simulink subsystem "encodersZ"  (R2023b)
settings: Solver=VariableStepAuto  StartTime=0.0  StopTime=10.0  RelTol=1e-3
libraries: arduinosensorlib x2, simulink x1
settings Model: Creator=Carlos  LastModifiedBy=Carlos

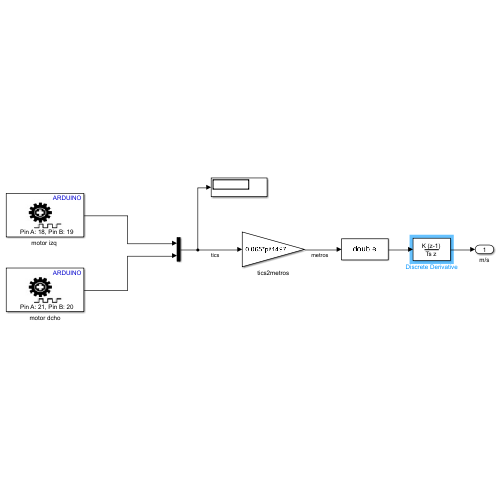
[thumbnail: Simulink's stored preview of the top-level diagram]
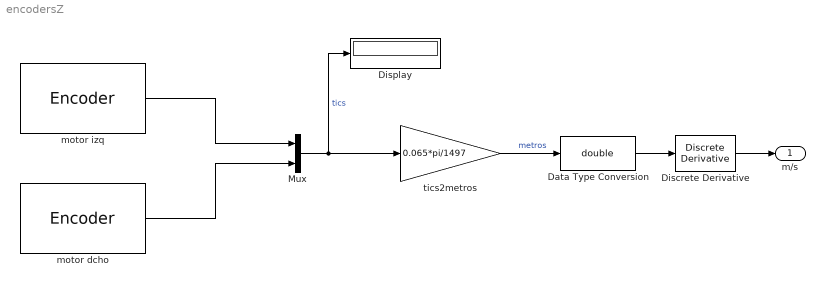
== system encodersZ ==
  Data Type Conversion : DataTypeConversion  OutDataTypeStr=double  SaturateOnIntegerOverflow=off  RndMeth=Floor
  Discrete Derivative : simulink/Discrete/Discrete Derivative  gainval=1.0  ICPrevScaledInput=0.0  OutMin=[]  OutMax=[]  OutDataType=fixdt(1, 16)  OutScaling=2^-10  DoSatur=off
  Display : Display
  Mux : Mux  Inputs=2
  motor dcho : arduinosensorlib/Encoder  InputA=21  InputB=20  Mode=No reset  SampleTime=-1
  "motor izq " : arduinosensorlib/Encoder  InputA=18  InputB=19  Mode=No reset  SampleTime=-1
  tics2metros : Gain  Gain=0.065*pi/1497
  m/s : Outport
  wires:
  tics2metros/1 -> Data Type Conversion/1  "metros"
  "motor izq "/1 -> Mux/1
  Mux/1 -> tics2metros/1, Display/1  "tics"
  motor dcho/1 -> Mux/2
  Data Type Conversion/1 -> Discrete Derivative/1
  Discrete Derivative/1 -> m/s/1
